simulink model "et_robocon_dev_guy"  (R2013b)
settings: Solver=FixedStepDiscrete  SolverMode=SingleTasking  StartTime=0.0  StopTime=inf  FixedStep=balancer_ts  RelTol=1e-3
undefined symbols (not defined in the file): a_d, a_r, balancerStates_Bus0, Batt, battery_gain, battery_offset, cmd_max, current_mode_status, current_task_operation_status, DiscIntNeverNeededParam, exec_period, Init_Bus0, k_f, k_i, k_phidot, k_thetadot, lightCalib, R, STATE, TRACK_MODE_LIST, ts2, W
libraries: simulink x29, legonxtlib x28, simulink_extras x4, light_sensor_calibration_algorithm_atomic_sub_chart_library x3, gyro_calibration_algorithm_atomic_sub_chart_library x1, limbo_algorithm_atomic_sub_chart_library x1, see_saw x1
(part 1 of 3)
settings Model: DataDictionary=mainDict.sldd  ExtModeTrigDuration=2  Creator=mbiesiad  LastModifiedBy=grouleau
settings ConfigSet: Description=Use this configuration to communicate between two robots. This robot is the master.
settings OptimizationCC: OptimizeModelRefInitCode=on  LifeSpan=1
settings DebuggingCC: UnderspecifiedInitializationDetection=Simplified  SolverPrmCheckMsg=none  ParameterPrecisionLossMsg=none  SignalLabelMismatchMsg=error  NonBusSignalsTreatedAsBus=error
settings HardwareCC: ProdLargestAtomicInteger=Long  ProdLargestAtomicFloat=Float  ProdEndianess=LittleEndian  ProdHWDeviceType=ARM Compatible->ARM 7
settings RTWCC: SystemTargetFile=realtime.tlc  GenerateMakefile=off  TemplateMakefile=realtime.tmf  Description=Run on Target Hardware  RTWVerbose=off  ProcessScript=realtime_make_rtw_hook
settings STFCustomTargetCC: TargetLibSuffix=.a  GenerateSampleERTMain=on  ERTCustomFileBanners=on  SupportNonInlinedSFcns=off  SupportVariableSizeSignals=on  MATLABClassNameForMDSCustomization=Simulink.SoftwareTarget.ERTCustomization  GRTInterface=off  SystemTargetFile=realtime.tlc
settings ERTTargetCC: CodeReplacementLibrary=ANSI_C  GenerateSampleERTMain=on  ParMdlRefBuildCompliant=off  CompOptLevelCompliant=off  ConcurrentExecutionCompliant=off  CombineOutputUpdateFcns=off  ERTFirstTimeCompliant=off  SupportContinuousTime=on  SupportVariableSizeSignals=on  ModelStepFunctionPrototypeControlCompliant=off  CPPClassGenCompliant=off  ExtModeTransport=1  ExtModeMexFile=ext_serial_win32_comm_no_acks_rtt_byteswap  ExtModeMexArgs=0 1 9600  InlinedParameterPlacement=NonHierarchical  ERTSrcFileBannerTemplate=realtime_code_template.cgt  ERTHdrFileBannerTemplate=realtime_code_template.cgt  ERTDataSrcFileTemplate=realtime_code_template.cgt  ERTDataHdrFileTemplate=realtime_code_template.cgt  ERTCustomFileTemplate=realtime_file_process.tlc

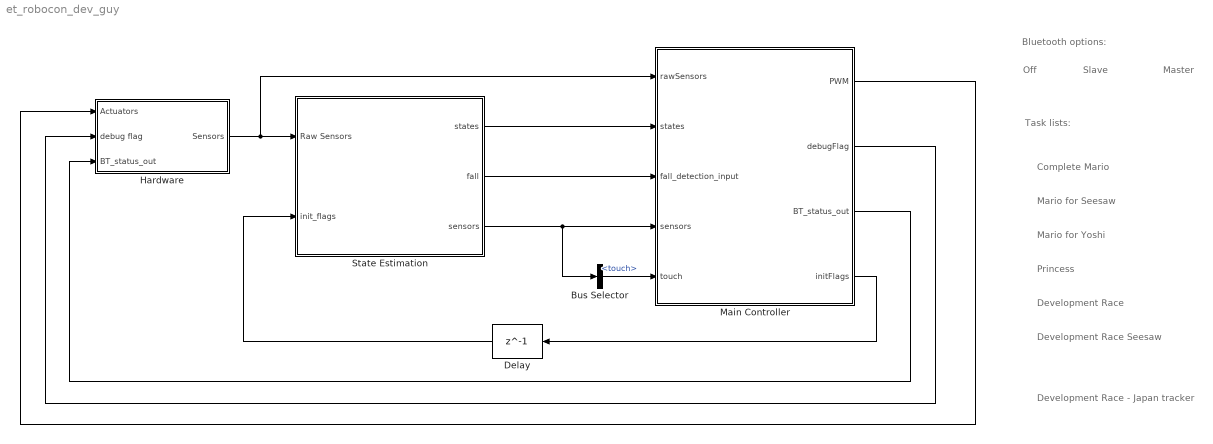
== system et_robocon_dev_guy ==
  note: Task lists:
  note: Bluetooth options:
  note: Slave
  note: Complete Mario
  note: Princess
  note: Mario for Seesaw
  note: Mario for Yoshi
  note: Development Race
  note: Development Race Seesaw
  note: Master
  note: Off
  note: Development Race - Japan tracker
  Bus Selector : BusSelector  OutputSignals=touch
  Delay : Delay  DelayLength=1
  Hardware : Subsystem  VariantControl=Variant1
  Main Controller : Stateflow chart  TreatAsAtomicUnit=on
  State Estimation : Subsystem
  wires:
  State Estimation/2(fall) -> Main Controller/3(fall_detection_input)
  State Estimation/3(sensors) -> Bus Selector/1, Main Controller/4(sensors)
  Bus Selector/1 -> Main Controller/5(touch)  "<touch>"
  Hardware/1(Sensors) -> Main Controller/1(rawSensors), State Estimation/1(Raw Sensors)
  Main Controller/4(initFlags) -> Delay/1
  State Estimation/1(states) -> Main Controller/2(states)
  Delay/1 -> State Estimation/2(init_flags)
  Main Controller/2(debugFlag) -> Hardware/2(debug flag)
  Main Controller/1(PWM) -> Hardware/1(Actuators)
  Main Controller/3(BT_status_out) -> Hardware/3(BT_status_out)

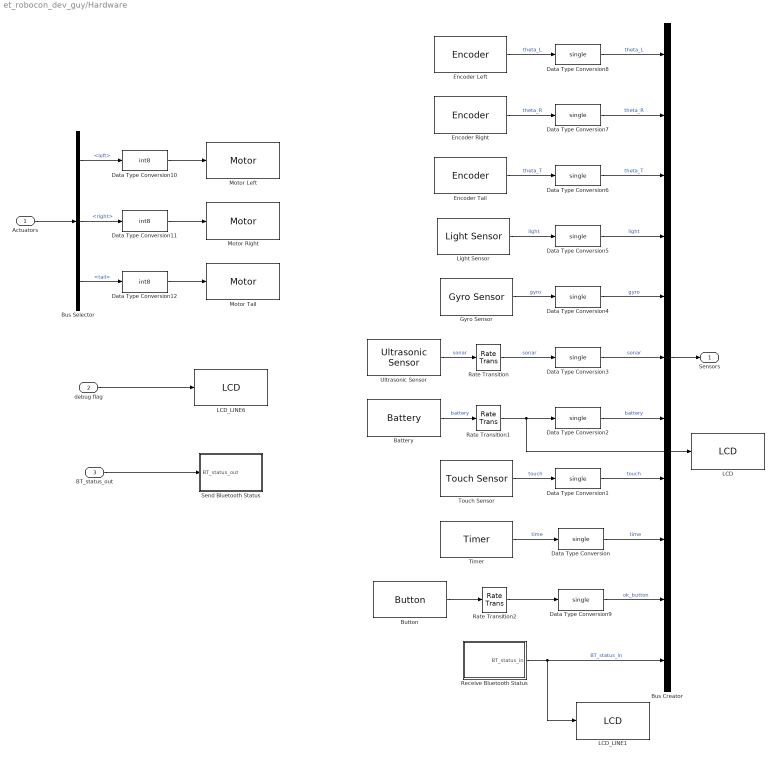
== system et_robocon_dev_guy/Hardware ==
  Actuators : Inport
  debug flag : Inport  Port=2
  BT_status_out : Inport  Port=3
  Battery : legonxtlib/Battery  sampleTime=.1
  Bus Creator : BusCreator  Inputs=11
  Bus Selector : BusSelector  OutputSignals=left,right,tail
  Button : legonxtlib/Button  buttonType=Middle orange  sampleTime=0.1
  Data Type Conversion{,1..9} (10 alike) : DataTypeConversion  OutDataTypeStr=single
  Data Type Conversion10 : DataTypeConversion  OutDataTypeStr=int8  SaturateOnIntegerOverflow=on
  Data Type Conversion11 : DataTypeConversion  OutDataTypeStr=int8  SaturateOnIntegerOverflow=on
  Data Type Conversion12 : DataTypeConversion  OutDataTypeStr=int8  SaturateOnIntegerOverflow=on
  Encoder Left : legonxtlib/Encoder  portNumber=C  opMode=No reset  sampleTime=0.004
  Encoder Right : legonxtlib/Encoder  portNumber=B  opMode=No reset  sampleTime=0.004
  Encoder Tail : legonxtlib/Encoder  portNumber=A  opMode=No reset  sampleTime=0.004
  Gyro Sensor : legonxtlib/Gyro Sensor  portNumber=1  outputMode=Raw A/D (0 - 1023)  offset=599  sampleTime=0.004
  LCD : legonxtlib/LCD  slcdStr=Batt:  slcdLine=3  slcdFormat=Decimal
  LCD_LINE1 : legonxtlib/LCD  slcdStr=BTSTATUS  slcdLine=2  slcdFormat=Decimal
  LCD_LINE6 : legonxtlib/LCD  slcdStr=STATE:  slcdLine=1  slcdFormat=Decimal
  Light Sensor : legonxtlib/Light Sensor  portNumber=3  outputMode=Raw A/D (1023 - 0)  lightOn=on  sampleTime=0.004
  Motor Left : legonxtlib/Motor  sportNumber=C  sstopAction=Brake
  Motor Right : legonxtlib/Motor  sportNumber=B  sstopAction=Brake
  Motor Tail : legonxtlib/Motor  sportNumber=A  sstopAction=Brake
  Rate Transition : RateTransition  OutPortSampleTime=0.004
  Rate Transition1 : RateTransition  OutPortSampleTime=0.004
  Rate Transition2 : RateTransition  OutPortSampleTime=0.004
  Receive Bluetooth Status : Subsystem  Variant=on
  Send Bluetooth Status : Subsystem  Variant=on
  Timer : legonxtlib/Timer  sampleTime=0.004
  Touch Sensor : legonxtlib/Touch Sensor  portNumber=4  sampleTime=0.004
  Ultrasonic Sensor : legonxtlib/Ultrasonic Sensor  PortNumber=2  sampleTime=0.02
  Sensors : Outport
  wires:
  Receive Bluetooth Status/1(BT_status_in) -> LCD_LINE1/1, Bus Creator/11  "BT_status_in"
  debug flag/1 -> LCD_LINE6/1
  Data Type Conversion9/1 -> Bus Creator/10  "ok_button"
  Rate Transition2/1 -> Data Type Conversion9/1
  Button/1 -> Rate Transition2/1
  Rate Transition1/1 -> LCD/1, Data Type Conversion2/1
  Data Type Conversion8/1 -> Bus Creator/1  "theta_L"
  Data Type Conversion7/1 -> Bus Creator/2  "theta_R"
  Data Type Conversion6/1 -> Bus Creator/3  "theta_T"
  Data Type Conversion5/1 -> Bus Creator/4  "light"
  Data Type Conversion4/1 -> Bus Creator/5  "gyro"
  Data Type Conversion3/1 -> Bus Creator/6  "sonar"
  Data Type Conversion2/1 -> Bus Creator/7  "battery"
  Data Type Conversion1/1 -> Bus Creator/8  "touch"
  Data Type Conversion/1 -> Bus Creator/9  "time"
  Rate Transition/1 -> Data Type Conversion3/1  "sonar"
  Ultrasonic Sensor/1 -> Rate Transition/1  "sonar"
  Bus Selector/3 -> Data Type Conversion12/1  "<tail>"
  Encoder Tail/1 -> Data Type Conversion6/1  "theta_T"
  Light Sensor/1 -> Data Type Conversion5/1  "light"
  Bus Selector/2 -> Data Type Conversion11/1  "<right>"
  Bus Selector/1 -> Data Type Conversion10/1  "<left>"
  Touch Sensor/1 -> Data Type Conversion1/1  "touch"
  Bus Creator/1 -> Sensors/1
  Battery/1 -> Rate Transition1/1  "battery"
  Gyro Sensor/1 -> Data Type Conversion4/1  "gyro"
  Encoder Right/1 -> Data Type Conversion7/1  "theta_R"
  Encoder Left/1 -> Data Type Conversion8/1  "theta_L"
  Timer/1 -> Data Type Conversion/1  "time"
  Actuators/1 -> Bus Selector/1
  Data Type Conversion10/1 -> Motor Left/1
  Data Type Conversion11/1 -> Motor Right/1
  Data Type Conversion12/1 -> Motor Tail/1
  BT_status_out/1 -> Send Bluetooth Status/1(BT_status_out)

== system et_robocon_dev_guy/Main Controller/normal_operation_modes.line_tracking_mode ==
  sensors : Inport
  touch : Inport  Port=2
  states : Inport  Port=3
  rawSensors : Inport  Port=4
  " Demux " : Demux
  " SFunction " : S-Function  Tag=Stateflow S-Function et_robocon_dev_guy 2  FunctionName=sf_sfun  PortCounts=[8 8]  EnableBusSupport=off
  line_tracking_mode.balanceControl : Subsystem
      settings: UndoDeleteFcn=Stateflow.SLINSF.SimulinkMan.restorePreDeleteFcn  PreDeleteFcn=Stateflow.SLINSF.SimulinkMan.removePreDeleteFcn
  line_tracking_mode.processLight : Subsystem
      settings: UndoDeleteFcn=Stateflow.SLINSF.SimulinkMan.restorePreDeleteFcn  PreDeleteFcn=Stateflow.SLINSF.SimulinkMan.removePreDeleteFcn
  line_tracking_mode.tail_controller : Subsystem
      settings: UndoDeleteFcn=Stateflow.SLINSF.SimulinkMan.restorePreDeleteFcn  PreDeleteFcn=Stateflow.SLINSF.SimulinkMan.removePreDeleteFcn
  line_tracking_mode.turnLightOn : Subsystem
      settings: UndoDeleteFcn=Stateflow.SLINSF.SimulinkMan.restorePreDeleteFcn  PreDeleteFcn=Stateflow.SLINSF.SimulinkMan.removePreDeleteFcn
  PWM : Outport
  debugFlag : Outport  Port=2
  wires:
  sensors/1 -> " SFunction "/1
  touch/1 -> " SFunction "/2
  states/1 -> " SFunction "/3
  rawSensors/1 -> " SFunction "/4
  " SFunction "/2 -> PWM/1  "PWM"
  " SFunction "/3 -> debugFlag/1  "debugFlag"
  " SFunction "/4 -> line_tracking_mode.processLight/1(rawSensors)
  line_tracking_mode.processLight/1(lineTrackCmd) -> " SFunction "/5
  " Demux "/1 -> line_tracking_mode.processLight/Trigger
  " SFunction "/5 -> line_tracking_mode.balanceControl/1(rawSensors)
  " SFunction "/6 -> line_tracking_mode.balanceControl/2(lineTrackCmd)
  line_tracking_mode.balanceControl/1(leftPWM) -> " SFunction "/6
  line_tracking_mode.balanceControl/2(rightPWM) -> " SFunction "/7
  " Demux "/2 -> line_tracking_mode.balanceControl/Trigger
  " SFunction "/7 -> line_tracking_mode.tail_controller/1(current)
  " SFunction "/8 -> line_tracking_mode.tail_controller/2(desired)
  line_tracking_mode.tail_controller/1(cmd) -> " SFunction "/8
  " Demux "/3 -> line_tracking_mode.tail_controller/Trigger
  " Demux "/4 -> line_tracking_mode.turnLightOn/Trigger
  " SFunction "/1 -> " Demux "/1

== system et_robocon_dev_guy/State Estimation ==
  Raw Sensors : Inport
  init_flags : Inport  Port=2
  Bus Selector1 : BusSelector  OutputSignals=tail,gyroInit,gyroReset,theta,fall
  Data Type Conversion Unit Conversion Tail Initialization : Subsystem
  Fall Detection : Subsystem
  Gyro Processing : Subsystem
  StateEstimation : Subsystem
  states : Outport
  fall : Outport  Port=2
  sensors : Outport  Port=3
  wires:
  Bus Selector1/3 -> Gyro Processing/3(gyroReset)  "<gyroReset>"
  Bus Selector1/4 -> StateEstimation/4(init theta)  "<theta>"
  Bus Selector1/1 -> Data Type Conversion Unit Conversion Tail Initialization/2(init_tail)  "<tail>"
  Bus Selector1/2 -> Gyro Processing/2(gyroInit)  "<gyroInit>"
  init_flags/1 -> Bus Selector1/1
  StateEstimation/1(states) -> states/1  "states"
  Data Type Conversion Unit Conversion Tail Initialization/1(y) -> sensors/1, StateEstimation/1(Sensors), Gyro Processing/1(sensors)
  Raw Sensors/1 -> Data Type Conversion Unit Conversion Tail Initialization/1(u)
  Gyro Processing/1(psi) -> StateEstimation/2(psi)
  Gyro Processing/2(psi_dot) -> StateEstimation/3(psi_dot)
  Gyro Processing/3(psi filtered) -> Fall Detection/1(gyro)
  Bus Selector1/5 -> Fall Detection/2(reset)  "<fall>"
  Fall Detection/1(fall_detected) -> fall/1

== system et_robocon_dev_guy/Hardware/Receive Bluetooth Status ==
  note: 1) Only subsystems can be added as variant choices at this level
      | 2) Blocks cannot be connected at this level as connectivity is
      | automatically determined at simulation, based on the active variant
  BluetoothOFF : Subsystem  VariantControl=BluetoothOFF
  BluetoothONMario : Subsystem  VariantControl=BluetoothONMario
  BluetoothONPrincess : Subsystem  VariantControl=BluetoothONPrincess
  BT_status_in : Outport

== system et_robocon_dev_guy/Hardware/Send Bluetooth Status ==
  note: 1) Only subsystems can be added as variant choices at this level
      | 2) Blocks cannot be connected at this level as connectivity is
      | automatically determined at simulation, based on the active variant
  BT_status_out : Inport
  BluetoothOFF : Subsystem  VariantControl=BluetoothOFF
  BluetoothONMario : Subsystem  VariantControl=BluetoothONMario
  BluetoothONPrincess : Subsystem  VariantControl=BluetoothONPrincess

== system et_robocon_dev_guy/Main Controller/normal_operation_modes.line_tracking_mode/line_tracking_mode.balanceControl ==
  rawSensors : Inport  OutDataTypeStr=Bus: Sensors_Bus  PortDimensions=1
  lineTrackCmd : Inport  Port=2  OutDataTypeStr=single  PortDimensions=2
  f : TriggerPort  TriggerType=function-call
      settings: CopyFcn=Stateflow.SLINSF.SimulinkMan.removeBlockPreDeleteFcn  PreDeleteFcn=Stateflow.SLINSF.SimulinkMan.unsafePredeleteFcn
  Bus Selector : BusSelector  OutputSignals=gyro,theta_L,theta_R,battery
  Constant3 : Constant  Value=612  OutDataTypeStr=uint16
  Data Type Conversion2 : DataTypeConversion  OutDataTypeStr=single  RndMeth=Simplest
      settings: AttributesFormatString=Round = %<RndMeth>
  Demux : Demux  Outputs=2
  ForSimulation : Subsystem  TreatAsAtomicUnit=on  RTWFcnName=balance_control  RTWFileName=balancer
      settings: RTWSystemCode=Nonreusable function  RTWFcnNameOpts=User specified  RTWFileNameOpts=User specified  FunctionWithSeparateData=on
  Low Pass Filter : Subsystem
  leftPWM : Outport  OutDataTypeStr=single  PortDimensions=1
  rightPWM : Outport  Port=2
  wires:
  ForSimulation/1(pwm_l) -> rightPWM/1
  ForSimulation/2(pwm_r) -> leftPWM/1
  rawSensors/1 -> Bus Selector/1
  lineTrackCmd/1 -> Demux/1
  Bus Selector/2 -> ForSimulation/5(theta_m_l)  "<theta_L>"
  Bus Selector/3 -> ForSimulation/6(theta_m_r)  "<theta_R>"
  Constant3/1 -> Data Type Conversion2/1
  Data Type Conversion2/1 -> ForSimulation/4(gyro_offset)  "gyro_offset"
  Bus Selector/1 -> ForSimulation/3(gyro)  "<gyro>"
  Bus Selector/4 -> Low Pass Filter/1(u)  "<battery>"
  Low Pass Filter/1(y) -> ForSimulation/7(battery)
  Demux/1 -> ForSimulation/1(cmd_forward)
  Demux/2 -> ForSimulation/2(cmd_turn)

== system et_robocon_dev_guy/Main Controller/normal_operation_modes.line_tracking_mode/line_tracking_mode.processLight ==
  rawSensors : Inport  OutDataTypeStr=Bus: Sensors_Bus  PortDimensions=1
  f : TriggerPort  TriggerType=function-call
      settings: CopyFcn=Stateflow.SLINSF.SimulinkMan.removeBlockPreDeleteFcn  PreDeleteFcn=Stateflow.SLINSF.SimulinkMan.unsafePredeleteFcn
  Bus Creator : BusCreator  Inputs=2
  Bus Creator2 : BusCreator  Inputs=2
  Bus Selector : BusSelector  OutputSignals=light,theta_R,theta_L,gyro
  Compare To Constant : simulink/Logic and Bit Operations/Compare To Constant  relop===  const=1  OutDataTypeStr=uint8
  Constant2 : Constant  Value=single(1)
  Constant3 : Constant  Value=612  OutDataTypeStr=uint16
  Data Store Memory18 : DataStoreMemory  DataStoreName=fwd_postmode_init  ReadBeforeWriteMsg=warning  WriteAfterWriteMsg=warning  WriteAfterReadMsg=warning
  Data Store Memory19 : DataStoreMemory  DataStoreName=fwd_premode_last  ReadBeforeWriteMsg=warning  WriteAfterWriteMsg=warning  WriteAfterReadMsg=warning
  Data Type Conversion2 : DataTypeConversion  OutDataTypeStr=single  RndMeth=Simplest
      settings: AttributesFormatString=Round = %<RndMeth>
  Filter : Subsystem
  LightOnOff : Subsystem
  LineTracePID : Subsystem  TreatAsAtomicUnit=on
      settings: RTWSystemCode=Nonreusable function
  MAP : Subsystem  TreatAsAtomicUnit=on
      settings: RTWSystemCode=Nonreusable function
  Signal Conversion : SignalConversion
  Signal Conversion1 : SignalConversion
  Unit Delay : UnitDelay  SampleTime=-1
  lineTrackCmd : Outport  OutDataTypeStr=single  PortDimensions=2  InitialOutput=[ 0 0]
  wires:
  rawSensors/1 -> Bus Selector/1
  LightOnOff/1(big) -> Filter/1(upped)
  Constant2/1 -> Compare To Constant/1
  Compare To Constant/1 -> LineTracePID/Enable
  Filter/2(centor) -> MAP/2(target)
  Filter/1(brightness) -> MAP/1(LightSens)
  MAP/1(LightSignal) -> LineTracePID/1(LightSens)  "LightSignal"
  LineTracePID/1(cmd) -> lineTrackCmd/1
  MAP/2(Brightness) -> LineTracePID/2(Brightness)
  LightOnOff/2(Small) -> Filter/2(dowened)
  Bus Creator/1 -> LineTracePID/3(EC)
  LineTracePID/2(bias) -> Unit Delay/1
  Unit Delay/1 -> Filter/3(bias1)
  Bus Creator2/1 -> LineTracePID/4(Gyro)
  Bus Selector/1 -> LightOnOff/1(RawLight)  "<light>"
  Bus Selector/2 -> Signal Conversion/1  "<theta_R>"
  Bus Selector/3 -> Signal Conversion1/1  "<theta_L>"
  Signal Conversion/1 -> Bus Creator/1  "R"
  Signal Conversion1/1 -> Bus Creator/2  "L"
  Constant3/1 -> Data Type Conversion2/1
  Data Type Conversion2/1 -> Bus Creator2/1  "gyro_offset"
  Bus Selector/4 -> Bus Creator2/2  "<gyro>"

== system et_robocon_dev_guy/Main Controller/normal_operation_modes.line_tracking_mode/line_tracking_mode.tail_controller ==
  note: Could be improved, PI for example
  current : Inport  OutDataTypeStr=single  PortDimensions=1
  desired : Inport  Port=2  OutDataTypeStr=single  PortDimensions=1
  f : TriggerPort  TriggerType=function-call
      settings: CopyFcn=Stateflow.SLINSF.SimulinkMan.removeBlockPreDeleteFcn  PreDeleteFcn=Stateflow.SLINSF.SimulinkMan.unsafePredeleteFcn
  Gain : Gain  Gain=250
  Saturation : Saturate  UpperLimit=100  LowerLimit=-100  OutDataTypeStr=single
  Sum : Sum  Inputs=|+-
  cmd : Outport  OutDataTypeStr=single  PortDimensions=1  InitialOutput=0
  wires:
  Sum/1 -> Gain/1
  current/1 -> Sum/2
  desired/1 -> Sum/1
  Gain/1 -> Saturation/1
  Saturation/1 -> cmd/1

== system et_robocon_dev_guy/Main Controller/normal_operation_modes.line_tracking_mode/line_tracking_mode.turnLightOn ==
  f : TriggerPort  TriggerType=function-call
      settings: CopyFcn=Stateflow.SLINSF.SimulinkMan.removeBlockPreDeleteFcn  PreDeleteFcn=Stateflow.SLINSF.SimulinkMan.unsafePredeleteFcn
  Light Sensor Switch ON : S-Function  FunctionName=sfun_light_sw  Parameters=-1,ip,sw  EnableBusSupport=off  mask(Light Sensor ON/OFF Switch){ip=S3, sw=ON}
      mask prompts: ip "port:"; sw "switch"
      mask help: LEGO Mindstorms NXT Light Sensor switch.
      mask init:
      | [data, map]=imread('LIGHT_SENSOR.gif');
      | pic=ind2rgb(data,map);
      mask TypeOptions ip: S1 | S2 | S3 | S4
      mask TypeOptions sw: ON | OFF
      mask Display:
      | image(pic)
      | color('red')
      | fprintf('%s, %s',ip,sw)

== system et_robocon_dev_guy/State Estimation/Data Type Conversion Unit Conversion Tail Initialization ==
  u : Inport
  init_tail : Inport  Port=2
  Bus Creator : BusCreator  Inputs=11  OutDataTypeStr=Bus: Sensors_Bus
  Bus Selector : BusSelector  OutputSignals=theta_L,theta_R,theta_T,light,gyro,sonar,battery,touch,time,ok_button,BT_status_in
  Degrees to Radians{,1..2,4} (4 alike) : simulink_extras/Transformations/Degrees to Radians
  Low Pass Filter : Subsystem
  Process Sonar : Subsystem  Commented=through
  Vmax : Subsystem
  tail processing : Subsystem
  y : Outport
  wires:
  Bus Selector/11 -> Bus Creator/11  "<BT_status_in>"
  Process Sonar/1(sonar) -> Bus Creator/6
  Bus Selector/6 -> Process Sonar/1(sonar_in)  "<sonar>"
  Bus Selector/10 -> Bus Creator/10  "<ok_button>"
  init_tail/1 -> tail processing/2(init_tail)
  Bus Selector/9 -> Bus Creator/9  "<time>"
  Bus Selector/8 -> Bus Creator/8  "<touch>"
  tail processing/1(tail) -> Bus Creator/3  "theta_T"
  Degrees to Radians4/1 -> tail processing/1(sensors)
  Vmax/1(Vmax) -> Bus Creator/7  "battery"
  Degrees to Radians2/1 -> Bus Creator/5  "gyro"
  Bus Selector/3 -> Degrees to Radians4/1  "<theta_T>"
  Bus Selector/7 -> Low Pass Filter/1(u)  "<battery>"
  Bus Selector/5 -> Degrees to Radians2/1  "<gyro>"
  Bus Selector/4 -> Bus Creator/4  "<light>"
  Bus Creator/1 -> y/1
  u/1 -> Bus Selector/1
  Degrees to Radians/1 -> Bus Creator/1  "theta_L"
  Bus Selector/2 -> Degrees to Radians1/1  "<theta_R>"
  Bus Selector/1 -> Degrees to Radians/1  "<theta_L>"
  Low Pass Filter/1(y) -> Vmax/1(Battery)  "battery"
  Degrees to Radians1/1 -> Bus Creator/2  "theta_R"

== system et_robocon_dev_guy/State Estimation/Fall Detection ==
  gyro : Inport
      settings: AttributesFormatString=Output data type: %<OutDataTypeStr>
  reset : Inport  Port=2  OutDataTypeStr=boolean
      settings: AttributesFormatString=Output data type: %<OutDataTypeStr>
  Abs : Abs
  Compare To Constant : simulink/Logic and Bit Operations/Compare To Constant  relop=>  const=1  OutDataTypeStr=boolean
  Terminator : Terminator
  aggregate_fall_detection_comparison : Logic  Operator=OR  OutDataTypeStr=boolean
  boolean_to_integer_conversion : DataTypeConversion  OutDataTypeStr=uint8
      settings: AttributesFormatString=Output data type: %<OutDataTypeStr>
  previous_fall_detection_status : UnitDelay  SampleTime=-1
  reset_output_overrice_switch : MultiPortSwitch  DataPortOrder=Zero-based contiguous  Inputs=2  zeroidx=on  InputSameDT=on
  reset_output_value : Constant  Value=false
  reset_output_value1 : Constant  Value=false  OutDataTypeStr=boolean
  fall_detected : Outport
  wires:
  reset_output_overrice_switch/1 -> Terminator/1, previous_fall_detection_status/1
  reset_output_value/1 -> reset_output_overrice_switch/3
  aggregate_fall_detection_comparison/1 -> reset_output_overrice_switch/2
  boolean_to_integer_conversion/1 -> reset_output_overrice_switch/1
  reset/1 -> boolean_to_integer_conversion/1
  previous_fall_detection_status/1 -> aggregate_fall_detection_comparison/2
  Abs/1 -> Compare To Constant/1
  gyro/1 -> Abs/1
  Compare To Constant/1 -> aggregate_fall_detection_comparison/1
  reset_output_value1/1 -> fall_detected/1

== system et_robocon_dev_guy/State Estimation/Gyro Processing ==
  sensors : Inport
  gyroInit : Inport  Port=2
  gyroReset : Inport  Port=3
  Bus Selector1 : BusSelector  OutputSignals=gyro
  Compute psi : Subsystem
  Gyro initialization : Subsystem  TreatAsAtomicUnit=on
  Reset Subsystem : Stateflow chart  TreatAsAtomicUnit=on
  Sum : Sum  Inputs=-+|
  psi : Outport
  psi_dot : Outport  Port=2
  psi filtered : Outport  Port=3
  wires:
  Compute psi/2(Filtered) -> psi filtered/1
  Reset Subsystem/1(doProcess()) -> Compute psi/Trigger
  gyroReset/1 -> Reset Subsystem/1(init_flag)
  Bus Selector1/1 -> Sum/2, Gyro initialization/1(gyro)  "<gyro>"
  Gyro initialization/1(psi_dot_0) -> Sum/1
  Sum/1 -> psi_dot/1, Compute psi/1(gyro)
  Compute psi/1(psi) -> psi/1
  sensors/1 -> Bus Selector1/1
  gyroInit/1 -> Gyro initialization/Enable

== system et_robocon_dev_guy/State Estimation/StateEstimation ==
  note: Conversion from Raw Sensors to States as described in "NXTway plant model.pdf"
  Sensors : Inport
  psi : Inport  Port=2
  psi_dot : Inport  Port=3
  init theta : Inport  Port=4
  Bus Creator1 : BusCreator  OutDataTypeStr=Bus: States_Bus
  Bus Creator2 : BusCreator  Inputs=5  OutDataTypeStr=Bus: Balancer_States_Bus
  Bus Selector1 : BusSelector  OutputSignals=theta_L,theta_R
  Process theta1 : Subsystem
  Reset Subsystem : Stateflow chart  TreatAsAtomicUnit=on
  states : Outport  OutputWhenDisabled=reset  InitialOutput=0
  wires:
  Process theta1/2(psi_out) -> Bus Creator2/2  "psi"
  Reset Subsystem/1(doProcess()) -> Process theta1/Trigger
  Bus Selector1/2 -> Process theta1/3(theta_r)  "<theta_R>"
  Bus Selector1/1 -> Process theta1/2(theta_l)  "<theta_L>"
  init theta/1 -> Reset Subsystem/1(init_flag)
  Process theta1/1(theta) -> Bus Creator2/1
  Process theta1/3(theta_dot) -> Bus Creator2/3
  Process theta1/4(int_theta) -> Bus Creator2/5
  psi_dot/1 -> Bus Creator2/4  "psi_dot"
  Process theta1/6(phi_dot) -> Bus Creator1/3  "phi_dot"
  Bus Creator2/1 -> Bus Creator1/1  "balancerStates"
  Process theta1/5(phi) -> Bus Creator1/2  "phi"
  Sensors/1 -> Bus Selector1/1
  psi/1 -> Process theta1/1(psi)
  Bus Creator1/1 -> states/1
  Process theta1/7(theta_dot_dot) -> Bus Creator1/4  "theta_dot_dot"

== system et_robocon_dev_guy/Hardware/Receive Bluetooth Status/BluetoothOFF ==
  Constant : Constant  Value=single(0)
  BT_status_in : Outport
  wires:
  Constant/1 -> BT_status_in/1

== system et_robocon_dev_guy/Hardware/Receive Bluetooth Status/BluetoothONMario ==
  Data Type Conversion9 : DataTypeConversion  OutDataTypeStr=single
  Rate Transition2 : RateTransition  OutPortSampleTime=0.004
  Receive via Bluetooth(R) Connection : legonxtlib/Receive via Bluetooth(R) Connection  mailbox=3  dataType=uint8  dataSize=1  sampleTime=0.1
  Terminator : Terminator
  BT_status_in : Outport
  wires:
  Data Type Conversion9/1 -> BT_status_in/1
  Rate Transition2/1 -> Data Type Conversion9/1
  Receive via Bluetooth(R) Connection/1 -> Rate Transition2/1
  Receive via Bluetooth(R) Connection/2 -> Terminator/1

== system et_robocon_dev_guy/Hardware/Receive Bluetooth Status/BluetoothONPrincess ==
  Data Type Conversion9 : DataTypeConversion  OutDataTypeStr=single
  Rate Transition2 : RateTransition  OutPortSampleTime=0.004
  Receive via Bluetooth(R) Connection : legonxtlib/Receive via Bluetooth(R) Connection  mailbox=2  dataType=uint8  dataSize=1  sampleTime=0.1
  Terminator : Terminator
  BT_status_in : Outport
  wires:
  Receive via Bluetooth(R) Connection/2 -> Terminator/1
  Receive via Bluetooth(R) Connection/1 -> Rate Transition2/1
  Rate Transition2/1 -> Data Type Conversion9/1
  Data Type Conversion9/1 -> BT_status_in/1

== system et_robocon_dev_guy/Hardware/Send Bluetooth Status/BluetoothOFF ==
  BT_status_out : Inport
  Terminator : Terminator
  wires:
  BT_status_out/1 -> Terminator/1

== system et_robocon_dev_guy/Hardware/Send Bluetooth Status/BluetoothONMario ==
  BT_status_out : Inport
  Data Type Conversion1 : DataTypeConversion  OutDataTypeStr=uint8
  Rate Transition1 : RateTransition  OutPortSampleTime=0.1
  Send via Bluetooth(R) Connection : legonxtlib/Send via Bluetooth(R) Connection  mailbox=2
  wires:
  BT_status_out/1 -> Rate Transition1/1
  Rate Transition1/1 -> Data Type Conversion1/1
  Data Type Conversion1/1 -> Send via Bluetooth(R) Connection/1

== system et_robocon_dev_guy/Hardware/Send Bluetooth Status/BluetoothONPrincess ==
  BT_status_out : Inport
  Data Type Conversion1 : DataTypeConversion  OutDataTypeStr=uint8
  Rate Transition1 : RateTransition  OutPortSampleTime=0.1
  Send via Bluetooth(R) Connection : legonxtlib/Send via Bluetooth(R) Connection  mailbox=3
  wires:
  Data Type Conversion1/1 -> Send via Bluetooth(R) Connection/1
  Rate Transition1/1 -> Data Type Conversion1/1
  BT_status_out/1 -> Rate Transition1/1

== system et_robocon_dev_guy/Main Controller/normal_operation_modes.line_tracking_mode/line_tracking_mode.balanceControl/ForSimulation ==
  cmd_forward : Inport
  cmd_turn : Inport  Port=2
  gyro : Inport  Port=3
  gyro_offset : Inport  Port=4
  theta_m_l : Inport  Port=5
  theta_m_r : Inport  Port=6
  battery : Inport  Port=7
  Cal_PWM : Subsystem
      settings: RTWSystemCode=Nonreusable function
  Cal_Reference : Subsystem  Description=|
      | 1111111111111111111
      | 2222222222222222222
      | 3333333333333333333
      | 4444444444444444444
      settings: RTWSystemCode=Nonreusable function
  Cal_x1 : Subsystem
      settings: RTWSystemCode=Nonreusable function
  DiscreteIntegrator : Subsystem
  FeedbackGain : Gain  Gain=k_f  Multiplication=Matrix(K*u)  OutDataTypeStr=Inherit: Same as input  ParamDataTypeStr=Inherit: Same as input
  IntegralGain : Gain  Gain=k_i  Multiplication=Matrix(K*u)  OutDataTypeStr=Inherit: Same as input  ParamDataTypeStr=Inherit: Same as input
  Sum1 : Sum  Inputs=|+-  OutDataTypeStr=Inherit: Same as first input
  Sum2 : Sum  Inputs=+-|  OutDataTypeStr=Inherit: Same as first input
  sum_err : Sum  Inputs=|++  OutDataTypeStr=Inherit: Same as first input
  pwm_l : Outport
  pwm_r : Outport  Port=2
  wires:
  Cal_Reference/1(pwm_turn) -> Cal_PWM/1(pwm_turn)
  cmd_turn/1 -> Cal_Reference/2(cmd_turn)
  sum_err/1 -> Cal_PWM/2(err)
  FeedbackGain/1 -> sum_err/2  "errx1"
  Cal_Reference/2(theta_ref) -> Sum1/1
  Cal_x1/1(theta) -> Sum1/2
  Sum1/1 -> DiscreteIntegrator/1(in)
  DiscreteIntegrator/1(out) -> IntegralGain/1
  IntegralGain/1 -> sum_err/1  "errtheta"
  Cal_x1/2(x1) -> Sum2/2
  Sum2/1 -> FeedbackGain/1
  Cal_Reference/3(x1_ref) -> Sum2/1
  theta_m_l/1 -> Cal_x1/3(theta_m_l)
  theta_m_r/1 -> Cal_x1/4(theta_m_r)
  cmd_forward/1 -> Cal_Reference/1(cmd_forward)
  Cal_PWM/1(pwm_l) -> pwm_l/1
  gyro/1 -> Cal_x1/1(gyro)
  Cal_PWM/2(pwm_r) -> pwm_r/1
  gyro_offset/1 -> Cal_x1/2(gyro_offset)
  battery/1 -> Cal_PWM/3(battery)

== system et_robocon_dev_guy/Main Controller/normal_operation_modes.line_tracking_mode/line_tracking_mode.balanceControl/Low Pass Filter ==
  u : Inport
  Constant : Constant  Value=0  OutDataTypeStr=boolean
  Low Pass Filter : DiscreteFilter  Numerator=[.01]  Denominator=[1 -0.99]
  Memory : Memory  X0=1  InheritSampleTime=on
  Store Offset : Subsystem  TreatAsAtomicUnit=on
  Sum1 : Sum  Inputs=++|
  Sum2 : Sum  Inputs=-+|
  y : Outport
  wires:
  Store Offset/1(x0) -> Sum1/1, Sum2/1
  u/1 -> Store Offset/1(x), Sum2/2
  Constant/1 -> Memory/1
  Memory/1 -> Store Offset/Enable
  Sum2/1 -> Low Pass Filter/1
  Sum1/1 -> y/1
  Low Pass Filter/1 -> Sum1/2

== system et_robocon_dev_guy/Main Controller/normal_operation_modes.line_tracking_mode/line_tracking_mode.processLight/Filter ==
  note: was -70
  note: was 85
  note: SlopeとStepの2箇所変更
  note: 95
  note: Output is always Zero for taraget (centor of Black and White)
  note: Light Sensor Filter Task
  upped : Inport
  dowened : Inport  Port=2
  bias1 : Inport  Port=3
  Ambient_Light_Rejection2 : Subsystem
  Constant1 : Constant  Value=70  OutDataTypeStr=single  SampleTime=-1
  Constant2 : Constant  Value=-50  OutDataTypeStr=single  SampleTime=-1
  LCD : legonxtlib/LCD  slcdStr=L  slcdLine=3  slcdFormat=Decimal
  Mux : Mux  Inputs=3
  Sum2 : Sum  Inputs=|++  OutDataTypeStr=single  RndMeth=Simplest
  bias5 : Constant  Value=0  OutDataTypeStr=single  SampleTime=-1
  brightness : Outport
  centor : Outport  Port=2
  wires:
  upped/1 -> Ambient_Light_Rejection2/1(Maximum)
  Constant2/1 -> Mux/1  "LightSens_Min"
  Constant1/1 -> Mux/3  "LightSens_Max"
  Mux/1 -> centor/1
  Sum2/1 -> Mux/2
  bias5/1 -> Sum2/1
  bias1/1 -> Sum2/2
  dowened/1 -> Ambient_Light_Rejection2/2(Minimum)
  Ambient_Light_Rejection2/1(Out1) -> LCD/1, brightness/1

== system et_robocon_dev_guy/Main Controller/normal_operation_modes.line_tracking_mode/line_tracking_mode.processLight/LightOnOff ==
  note: Light sensor ON/OFF control
  note: Light sensor ON/OFF control Task
  RawLight : Inport
  Constant2 : Constant  OutDataTypeStr=uint8
  Constant4 : Constant  Value=0  OutDataTypeStr=uint8
  OFF2ON : Subsystem  TreatAsAtomicUnit=on
  ON2OFF : Subsystem  TreatAsAtomicUnit=on
  Switch : Switch  Threshold=0.5
  Unit Delay2 : UnitDelay  SampleTime=-1
  big : Outport
  Small : Outport  Port=2
  wires:
  Unit Delay2/1 -> Switch/2
  Constant4/1 -> Switch/1
  Constant2/1 -> Switch/3
  Switch/1 -> Unit Delay2/1, OFF2ON/Trigger, ON2OFF/Trigger
  RawLight/1 -> ON2OFF/1(In1), OFF2ON/1(In1)
  OFF2ON/1(Out1) -> big/1
  ON2OFF/1(Out1) -> Small/1

== system et_robocon_dev_guy/Main Controller/normal_operation_modes.line_tracking_mode/line_tracking_mode.processLight/LineTracePID ==
  note: This signal seems to come from BT in original,
      | but because I have have no idea what it should be I will plug a zero... to clarify
      | Inwhat we sa, I think there was no BT, so my best guess is that zero was used
  note: Output is string for Balance library.
  note: Light Tracking PID control Task
  LightSens : Inport
  Brightness : Inport  Port=2
  EC : Inport  Port=3
  Gyro : Inport  Port=4
  Enable : EnablePort  StatesWhenEnabling=reset
  AngleCounter : Subsystem
  Constant4 : Constant  Value=0  OutDataTypeStr=single  SampleTime=-1
  Data Store Write2 : DataStoreWrite  DataStoreName=fwd_premode_last
  Handler : Subsystem
  Signal Conversion : SignalConversion
  SwitchController : Subsystem  TreatAsAtomicUnit=on
  SwutchForFreeSteering : Subsystem
  cmd : Outport  InitialOutput=[0 0]
  bias : Outport  Port=2  InitialOutput=0
  wires:
  Handler/1(Out1) -> cmd/1
  Constant4/1 -> Handler/3(sw)
  EC/1 -> AngleCounter/1(EC)
  AngleCounter/1(AngleCount) -> SwitchController/1(Cnt)
  Brightness/1 -> SwitchController/4(LigthSens)
  Gyro/1 -> SwitchController/5(Gyro)
  SwitchController/4(bias) -> bias/1
  AngleCounter/2(EncoderReseted) -> SwitchController/2(EC_reseted)
  AngleCounter/3(Angle) -> SwitchController/3(Angle)
  SwitchController/3(fwd) -> Signal Conversion/1, Handler/2(fwd)
  SwitchController/1(Flag_steering) -> SwutchForFreeSteering/1(FlagSteering)
  SwitchController/2(PID) -> SwutchForFreeSteering/2(PID)
  LightSens/1 -> SwutchForFreeSteering/3(LightSens)
  SwutchForFreeSteering/1(Steering) -> Handler/1(steering)
  Signal Conversion/1 -> Data Store Write2/1

== system et_robocon_dev_guy/Main Controller/normal_operation_modes.line_tracking_mode/line_tracking_mode.processLight/MAP ==
  note: 110
  note: 280
  note: 70
  note: 240
  note: circle
  note: bias
  note: 65
  note: 220
  note: real
  note: Output is between Zero (white) to One (Black).
  note: Light Sensor MAP Task
  LightSens : Inport
  target : Inport  Port=2
  Constant3 : Constant  Value=[0, 0.5, 1]  OutDataTypeStr=single  SampleTime=-1
  Data Type Conversion2 : DataTypeConversion  OutDataTypeStr=single  RndMeth=Simplest
      settings: AttributesFormatString=Round = %<RndMeth>
  Lookup Table Dynamic : simulink/Lookup Tables/Lookup Table Dynamic  LookUpMeth=Interpolation-Use End Values  OutDataTypeStr=fixdt('single')  OutputDataTypeScalingMode=Specify via dialog  OutDataType=fixdt('single')  OutScaling=[]  RndMeth=Simplest  DoSatur=off
  LightSignal : Outport
  Brightness : Outport  Port=2
  wires:
  Data Type Conversion2/1 -> Lookup Table Dynamic/2
  Constant3/1 -> Lookup Table Dynamic/3
  Lookup Table Dynamic/1 -> LightSignal/1
  target/1 -> Data Type Conversion2/1
  LightSens/1 -> Lookup Table Dynamic/1, Brightness/1

== system et_robocon_dev_guy/State Estimation/Data Type Conversion Unit Conversion Tail Initialization/Low Pass Filter ==
  u : Inport
  Constant : Constant  Value=0  OutDataTypeStr=boolean
  Low Pass Filter : DiscreteFilter  Numerator=[.01]  Denominator=[1 -0.99]
  Memory : Memory  X0=1  InheritSampleTime=on
  Store Offset : Subsystem  TreatAsAtomicUnit=on
  Sum1 : Sum  Inputs=++|
  Sum2 : Sum  Inputs=-+|
  y : Outport
  wires:
  Store Offset/1(x0) -> Sum1/1, Sum2/1
  u/1 -> Store Offset/1(x), Sum2/2
  Constant/1 -> Memory/1
  Memory/1 -> Store Offset/Enable
  Sum2/1 -> Low Pass Filter/1
  Sum1/1 -> y/1
  Low Pass Filter/1 -> Sum1/2

== system et_robocon_dev_guy/State Estimation/Data Type Conversion Unit Conversion Tail Initialization/Process Sonar ==
  sonar_in : Inport
  Constant : Constant  Value=single(255)
  Logical Operator : Logic  Inputs=4  AllPortsSameDT=off  OutDataTypeStr=boolean
  Logical Operator1 : Logic  Operator=NOT  AllPortsSameDT=off  OutDataTypeStr=boolean
  Rate Transition : RateTransition  OutPortSampleTime=0.02
  Rate Transition1 : RateTransition  OutPortSampleTime=0.004
  Relational Operator{,1..3} (4 alike) : RelationalOperator  Operator===  OutDataTypeStr=boolean
  Switch : Switch  Criteria=u2 ~= 0
  Unit Delay{,1..3} (4 alike) : UnitDelay  SampleTime=-1
  sonar : Outport
  wires:
  Switch/1 -> sonar/1  "sonar"
  Constant/1 -> Switch/3
  Rate Transition1/1 -> Switch/2
  Logical Operator1/1 -> Rate Transition1/1
  Logical Operator/1 -> Logical Operator1/1
  Relational Operator2/1 -> Logical Operator/3
  Relational Operator1/1 -> Logical Operator/2
  Relational Operator3/1 -> Logical Operator/4
  Relational Operator/1 -> Logical Operator/1
  Unit Delay3/1 -> Relational Operator3/2
  Unit Delay2/1 -> Unit Delay3/1, Relational Operator2/2, Relational Operator3/1
  Unit Delay1/1 -> Unit Delay2/1, Relational Operator1/2, Relational Operator2/1
  Unit Delay/1 -> Unit Delay1/1, Relational Operator/2, Relational Operator1/1
  Rate Transition/1 -> Unit Delay/1, Relational Operator/1
  sonar_in/1 -> Rate Transition/1, Switch/1

== system et_robocon_dev_guy/State Estimation/Data Type Conversion Unit Conversion Tail Initialization/Vmax ==
  Battery : Inport
  Constant : Constant  Value=0.625  OutDataTypeStr=single
  Gain1 : Gain  Gain=0.001089
  Sum : Sum  Inputs=|+-
  Vmax : Outport
  wires:
  Battery/1 -> Gain1/1
  Gain1/1 -> Sum/1
  Constant/1 -> Sum/2
  Sum/1 -> Vmax/1

== system et_robocon_dev_guy/State Estimation/Data Type Conversion Unit Conversion Tail Initialization/tail processing ==
  sensors : Inport
  init_tail : Inport  Port=2
  Sum : Sum  Inputs=-+|
  tail initialization : Subsystem  TreatAsAtomicUnit=on
  tail : Outport  OutputWhenDisabled=reset  InitialOutput=0
  wires:
  Sum/1 -> tail/1  "theta_T"
  sensors/1 -> Sum/2, tail initialization/1(tail)
  tail initialization/1(tail_0) -> Sum/1
  init_tail/1 -> tail initialization/Trigger

== system et_robocon_dev_guy/State Estimation/Gyro Processing/Compute psi ==
  gyro : Inport
  Trigger : TriggerPort  TriggerType=function-call  StatesWhenEnabling=reset  PortDimensions=1
  Discrete-Time Integrator : DiscreteIntegrator  SampleTime=-1  ICPrevOutput=DiscIntNeverNeededParam  ICPrevScaledInput=DiscIntNeverNeededParam
  Discrete-Time Integrator1 : DiscreteIntegrator  SampleTime=-1  ICPrevOutput=DiscIntNeverNeededParam  ICPrevScaledInput=DiscIntNeverNeededParam
  Sum3 : Sum  Inputs=|+-
  Very Low Pass Filter : Subsystem
  psi : Outport  InitialOutput=0
  Filtered : Outport  Port=2  InitialOutput=0
  wires:
  Discrete-Time Integrator/1 -> Filtered/1
  Discrete-Time Integrator1/1 -> psi/1
  Sum3/1 -> Discrete-Time Integrator/1
  Very Low Pass Filter/1(Out1) -> Sum3/2
  gyro/1 -> Very Low Pass Filter/1(In1), Sum3/1, Discrete-Time Integrator1/1

== system et_robocon_dev_guy/State Estimation/Gyro Processing/Gyro initialization ==
  gyro : Inport
  Enable : EnablePort  StatesWhenEnabling=reset
  Low Pass Filter : DiscreteFilter  Numerator=[.01]  Denominator=[1 -0.99]
  psi_dot_0 : Outport  InitialOutput=0
  wires:
  Low Pass Filter/1 -> psi_dot_0/1
  gyro/1 -> Low Pass Filter/1

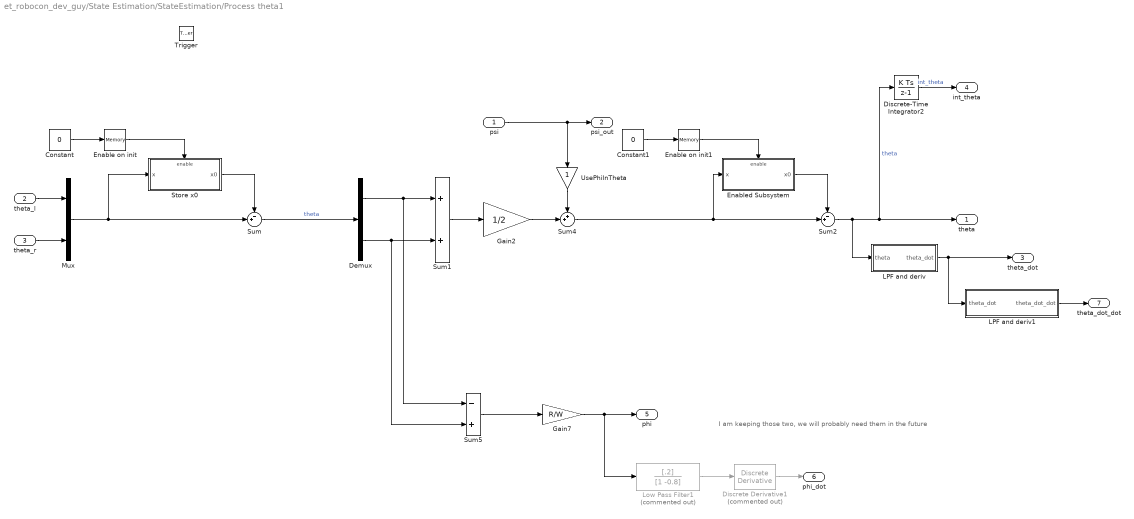
== system et_robocon_dev_guy/State Estimation/StateEstimation/Process theta1 ==
  note: I am keeping those two, we will probably need them in the future
  psi : Inport
  theta_l : Inport  Port=2
  theta_r : Inport  Port=3
  Trigger : TriggerPort  TriggerType=function-call  StatesWhenEnabling=reset  PortDimensions=1
  Constant : Constant  Value=0  OutDataTypeStr=boolean
  Constant1 : Constant  Value=0  OutDataTypeStr=boolean
  Demux : Demux  Outputs=2
  Discrete Derivative1 : simulink/Discrete/Discrete Derivative  Commented=on  gainval=1.0  ICPrevScaledInput=0.0  InputProcessing=Inherited  OutMin=[]  OutMax=[]  OutDataType=fixdt(1, 16)  OutScaling=2^-10  DoSatur=off
  Discrete-Time Integrator2 : DiscreteIntegrator  SampleTime=-1  ICPrevOutput=DiscIntNeverNeededParam  ICPrevScaledInput=DiscIntNeverNeededParam
  Enable on init : Memory  X0=1  InheritSampleTime=on
  Enable on init1 : Memory  X0=1  InheritSampleTime=on
  Enabled Subsystem : Subsystem  TreatAsAtomicUnit=on
  Gain2 : Gain  Gain=1/2
  Gain7 : Gain  Gain=R/W
  LPF and deriv : Subsystem
  LPF and deriv1 : Subsystem
  Low Pass Filter1 : DiscreteFilter  Commented=on  Numerator=[.2]  Denominator=[1 -0.8]
  Mux : Mux  Inputs=2
  Store x0 : Subsystem  TreatAsAtomicUnit=on
  Sum : Sum  Inputs=-+|
  Sum1 : Sum
  Sum2 : Sum  Inputs=-+|
  Sum4 : Sum  Inputs=++|
  Sum5 : Sum  Inputs=-+
  UsePhiInTheta : Gain
  theta : Outport  InitialOutput=0
  psi_out : Outport  Port=2  InitialOutput=0
  theta_dot : Outport  Port=3  OutputWhenDisabled=reset  InitialOutput=0
  int_theta : Outport  Port=4  InitialOutput=0
  phi : Outport  Port=5  OutputWhenDisabled=reset  InitialOutput=0
  phi_dot : Outport  Port=6  OutputWhenDisabled=reset  InitialOutput=0
  theta_dot_dot : Outport  Port=7  OutputWhenDisabled=reset  InitialOutput=0
  wires:
  Gain7/1 -> Low Pass Filter1/1, phi/1
  Sum5/1 -> Gain7/1
  Sum2/1 -> LPF and deriv/1(theta), theta/1, Discrete-Time Integrator2/1  "theta"
  Enabled Subsystem/1(x0) -> Sum2/1
  Constant1/1 -> Enable on init1/1
  Enable on init1/1 -> Enabled Subsystem/Enable
  Sum4/1 -> Sum2/2, Enabled Subsystem/1(x)
  Discrete-Time Integrator2/1 -> int_theta/1  "int_theta"
  psi/1 -> UsePhiInTheta/1, psi_out/1
  UsePhiInTheta/1 -> Sum4/1
  Sum1/1 -> Gain2/1
  Gain2/1 -> Sum4/2
  Demux/2 -> Sum1/2, Sum5/2
  Demux/1 -> Sum1/1, Sum5/1
  theta_r/1 -> Mux/2
  theta_l/1 -> Mux/1
  Mux/1 -> Sum/2, Store x0/1(x)
  Sum/1 -> Demux/1  "theta"
  Store x0/1(x0) -> Sum/1
  Constant/1 -> Enable on init/1
  Enable on init/1 -> Store x0/Enable
  Low Pass Filter1/1 -> Discrete Derivative1/1
  Discrete Derivative1/1 -> phi_dot/1
  LPF and deriv/1(theta_dot) -> LPF and deriv1/1(theta_dot), theta_dot/1
  LPF and deriv1/1(theta_dot_dot) -> theta_dot_dot/1

== system et_robocon_dev_guy/Main Controller/normal_operation_modes.line_tracking_mode/line_tracking_mode.balanceControl/ForSimulation/Cal_PWM ==
  note: Calculate maximum of DC motor
      | voltatege from battery using an
      | experimental expression.
  note: Turn NXTway-GS by applying pwm offset
      | to left and right motor in the counter direction.
  pwm_turn : Inport
  err : Inport  Port=2
  battery : Inport  Port=3
  Cal_vol_max : Subsystem
  Gain : Gain  Gain=100  OutDataTypeStr=Inherit: Same as input  ParamDataTypeStr=Inherit: Same as input
  Product : Product  Inputs=*/  RndMeth=Simplest  OutDataTypeStr=Inherit: Same as first input
  Sum : Sum  Inputs=|++  OutDataTypeStr=Inherit: Same as first input
  Sum1 : Sum  Inputs=|+-  OutDataTypeStr=Inherit: Same as first input
  pwm_l_limiter : Saturate  UpperLimit=100  LowerLimit=-100
      settings: AttributesFormatString=max = %<UpperLimit>\nmin = %<LowerLimit>
  pwm_r_limiter : Saturate  UpperLimit=100  LowerLimit=-100
      settings: AttributesFormatString=max = %<UpperLimit>\nmin = %<LowerLimit>
  pwm_l : Outport
  pwm_r : Outport  Port=2
  wires:
  Sum/1 -> pwm_l_limiter/1
  pwm_turn/1 -> Sum/2, Sum1/2
  Gain/1 -> Sum1/1, Sum/1
  err/1 -> Product/1
  Product/1 -> Gain/1
  battery/1 -> Cal_vol_max/1(battery)
  Cal_vol_max/1(vol_max) -> Product/2
  Sum1/1 -> pwm_r_limiter/1
  pwm_r_limiter/1 -> pwm_r/1
  pwm_l_limiter/1 -> pwm_l/1

== system et_robocon_dev_guy/Main Controller/normal_operation_modes.line_tracking_mode/line_tracking_mode.balanceControl/ForSimulation/Cal_Reference ==
  note: Divide command values by
      | maximum of command input.
  note: Smooth velocity command
      | using Low Path Filter to
      | suppress rapid input change.
  cmd_forward : Inport
  cmd_turn : Inport  Port=2
  Constant1 : Constant  Value=cmd_max  VectorParams1D=off  OutDataTypeStr=single  SampleTime=-1
      settings: AttributesFormatString=DataType = %<OutDataTypeStr>
  Constant2 : Constant  Value=0  VectorParams1D=off  OutDataTypeStr=single  SampleTime=-1
      settings: AttributesFormatString=DataType = %<OutDataTypeStr>
  Constant3 : Constant  Value=0  VectorParams1D=off  OutDataTypeStr=single  SampleTime=-1
      settings: AttributesFormatString=DataType = %<OutDataTypeStr>
  Constant6 : Constant  Value=cmd_max  VectorParams1D=off  OutDataTypeStr=single  SampleTime=-1
      settings: AttributesFormatString=DataType = %<OutDataTypeStr>
  DiscreteIntegrator : Subsystem
  Divide : Product  Inputs=*/  RndMeth=Simplest  OutDataTypeStr=Inherit: Same as first input
  Divide1 : Product  Inputs=*/  RndMeth=Simplest  OutDataTypeStr=Inherit: Same as first input
  Gain1 : Gain  Gain=k_thetadot  OutDataTypeStr=Inherit: Same as input  ParamDataTypeStr=Inherit: Same as input
  Gain2 : Gain  Gain=k_phidot  OutDataTypeStr=Inherit: Same as input  ParamDataTypeStr=Inherit: Same as input
  LowPathFilter : Subsystem
  Mux : Mux
  pwm_turn : Outport
  theta_ref : Outport  Port=2
  x1_ref : Outport  Port=3
  wires:
  cmd_turn/1 -> Divide1/1
  Gain1/1 -> LowPathFilter/1(in)
  cmd_forward/1 -> Divide/1
  Divide/1 -> Gain1/1
  Gain2/1 -> pwm_turn/1  "pwm_turn"
  Constant1/1 -> Divide1/2
  Divide1/1 -> Gain2/1
  Mux/1 -> x1_ref/1
  DiscreteIntegrator/1(out) -> theta_ref/1, Mux/1  "theta_ref"
  Constant2/1 -> Mux/2  "psi_ref"
  Constant3/1 -> Mux/4  "psidot_ref"
  LowPathFilter/1(out) -> Mux/3, DiscreteIntegrator/1(in)  "thetadot_ref"
  Constant6/1 -> Divide/2

== system et_robocon_dev_guy/Main Controller/normal_operation_modes.line_tracking_mode/line_tracking_mode.balanceControl/ForSimulation/Cal_x1 ==
  note: Smooth measured velocity value using
      | Low Path Filter to reduce the noise
      | because it makes extra control input.
  note: Calculate gyro offset for removing gyro drift.
  gyro : Inport
  gyro_offset : Inport  Port=2
  theta_m_l : Inport  Port=3
  theta_m_r : Inport  Port=4
  DiscreteDerivative : Subsystem
  DiscreteIntegrator : Subsystem
  Gain : Gain  Gain=1/2  OutDataTypeStr=Inherit: Same as input  ParamDataTypeStr=Inherit: Same as input
  LowPathFilter : Subsystem
  Mux1 : Mux
  Sum1 : Sum  Inputs=++|  OutDataTypeStr=Inherit: Same as first input
  Sum2 : Sum  Inputs=|+-  OutDataTypeStr=Inherit: Same as first input
  Sum4 : Sum  Inputs=|++  OutDataTypeStr=Inherit: Same as first input
  Sum6 : Sum  Inputs=|++  OutDataTypeStr=Inherit: Same as first input
  deg2rad : Gain  Gain=deg2rad  OutDataTypeStr=Inherit: Same as input  ParamDataTypeStr=Inherit: Same as input
  deg2rad1 : Gain  Gain=deg2rad  OutDataTypeStr=Inherit: Same as input  ParamDataTypeStr=Inherit: Same as input
  deg2rad2 : Gain  Gain=deg2rad  OutDataTypeStr=Inherit: Same as input  ParamDataTypeStr=Inherit: Same as input
  theta : Outport
  x1 : Outport  Port=2
  wires:
  deg2rad1/1 -> Sum4/1
  Mux1/1 -> x1/1
  DiscreteIntegrator/1(out) -> Sum6/2, Sum4/2, Mux1/2  "psi"
  deg2rad/1 -> Sum6/1
  theta_m_l/1 -> deg2rad/1
  theta_m_r/1 -> deg2rad1/1
  DiscreteDerivative/1(out) -> Mux1/3  "thetadot"
  Sum6/1 -> Sum1/1  "theta_l"
  Sum4/1 -> Sum1/2  "theta_r"
  Sum1/1 -> Gain/1  "thata_m_sum"
  gyro/1 -> Sum2/1
  Sum2/1 -> deg2rad2/1
  deg2rad2/1 -> Mux1/4, DiscreteIntegrator/1(in)  "psidot"
  LowPathFilter/1(out) -> DiscreteDerivative/1(in)
  Gain/1 -> theta/1, Mux1/1, LowPathFilter/1(in)  "theta"
  gyro_offset/1 -> Sum2/2
  LowPathFilter/2(out1) -> DiscreteDerivative/2(in1)

== system et_robocon_dev_guy/Main Controller/normal_operation_modes.line_tracking_mode/line_tracking_mode.balanceControl/ForSimulation/DiscreteIntegrator ==
  in : Inport
  Gain : Gain  Gain=exec_period  OutDataTypeStr=Inherit: Same as input  ParamDataTypeStr=Inherit: Same as input
  Sum : Sum  Inputs=|++  OutDataTypeStr=Inherit: Same as first input
  Unit Delay : UnitDelay  SampleTime=-1  StateName=ud_psi  StateMustResolveToSignalObject=on
      settings: AttributesFormatString=Signal name = ud_psi
  out : Outport
  wires:
  Unit Delay/1 -> Sum/2, out/1
  Gain/1 -> Sum/1
  Sum/1 -> Unit Delay/1
  in/1 -> Gain/1

== system et_robocon_dev_guy/Main Controller/normal_operation_modes.line_tracking_mode/line_tracking_mode.balanceControl/Low Pass Filter/Store Offset ==
  x : Inport
  Enable : EnablePort
  x0 : Outport  InitialOutput=0
  wires:
  x/1 -> x0/1

== system et_robocon_dev_guy/Main Controller/normal_operation_modes.line_tracking_mode/line_tracking_mode.processLight/Filter/Ambient_Light_Rejection2 ==
  Maximum : Inport
  Minimum : Inport  Port=2
  Constant : Constant  Value=0  OutDataTypeStr=single  SampleTime=-1
  Gain : Gain  Gain=0.004736
  Gain1 : Gain  Gain=3.295
  Gain2 : Gain  Gain=0.0002337
  Gain3 : Gain  Gain=-15.78
  Math Function : Math  SaturateOnIntegerOverflow=on
  Math Function1 : Math  SaturateOnIntegerOverflow=on
  Sum1 : Sum  Inputs=+-|
  Sum2 : Sum  Inputs=|+-
  Sum3 : Sum  Inputs=|++
  Switch : Switch  Criteria=u2 > Threshold  RndMeth=Simplest
  Out1 : Outport
  wires:
  Switch/1 -> Sum2/2
  Sum3/1 -> Sum2/1
  Gain3/1 -> Sum3/2
  Gain1/1 -> Sum3/1
  Math Function1/1 -> Gain3/1
  Gain2/1 -> Math Function1/1
  Sum1/1 -> Switch/2, Switch/1
  Constant/1 -> Switch/3
  Math Function/1 -> Gain1/1
  Gain/1 -> Math Function/1
  Maximum/1 -> Gain2/1, Sum1/1, Gain/1
  Sum2/1 -> Out1/1
  Minimum/1 -> Sum1/2

== system et_robocon_dev_guy/Main Controller/normal_operation_modes.line_tracking_mode/line_tracking_mode.processLight/LightOnOff/OFF2ON ==
  In1 : Inport
  Trigger : TriggerPort
  Light Sensor Switch ON : S-Function  FunctionName=sfun_light_sw  Parameters=-1,ip,sw  EnableBusSupport=off  mask(Light Sensor ON/OFF Switch){ip=S3, sw=ON}
      mask prompts: ip "port:"; sw "switch"
      mask help: LEGO Mindstorms NXT Light Sensor switch.
      mask init:
      | [data, map]=imread('LIGHT_SENSOR.gif');
      | pic=ind2rgb(data,map);
      mask TypeOptions ip: S1 | S2 | S3 | S4
      mask TypeOptions sw: ON | OFF
      mask Display:
      | image(pic)
      | color('red')
      | fprintf('%s, %s',ip,sw)
  Out1 : Outport
  wires:
  In1/1 -> Out1/1

== system et_robocon_dev_guy/Main Controller/normal_operation_modes.line_tracking_mode/line_tracking_mode.processLight/LightOnOff/ON2OFF ==
  In1 : Inport
  Trigger : TriggerPort  TriggerType=falling
  Light Sensor Switch OFF : S-Function  FunctionName=sfun_light_sw  Parameters=-1,ip,sw  EnableBusSupport=off  mask(Light Sensor ON/OFF Switch){ip=S3, sw=OFF}
      mask prompts: ip "port:"; sw "switch"
      mask help: LEGO Mindstorms NXT Light Sensor switch.
      mask init:
      | [data, map]=imread('LIGHT_SENSOR.gif');
      | pic=ind2rgb(data,map);
      mask TypeOptions ip: S1 | S2 | S3 | S4
      mask TypeOptions sw: ON | OFF
      mask Display:
      | image(pic)
      | color('red')
      | fprintf('%s, %s',ip,sw)
  Out1 : Outport
  wires:
  In1/1 -> Out1/1
